simulink model "labsetup_cantonisim_distributed_periodic"  (R2019a)
settings: Solver=FixedStepDiscrete  StartTime=0.0  StopTime=1000  FixedStep=h  RelTol=1e-3
InitFcn:
  | ini_cantonisim_distributed
values from neighbouring files (symbols this model uses):
  C1 = [1 0]    [cantoni_LMI_labsetup.m]    (also in distributed_workspace_bak.mat)
  C2 = [0 1]    [cantoni_LMI_labsetup.m]    (also in distributed_workspace_bak.mat)
  ddelay = [0 0]    [distributed_workspace_bak.mat]
  h = legend(strcat('\phi(',plantTitle,')')); set(h,'FontSize',18)    [bodeJL.m]    (also in cantoni_LMI_labsetup.m = 1; distributed_workspace_bak.mat = 1)
  P1d = c2d(P1, h, 'zoh')    [cantoni_LMI_labsetup.m]
  P2d = c2d(P2, h, 'zoh')    [cantoni_LMI_labsetup.m]
  ss1d = c2d(ss1, h, 'tustin')    [cantoni_LMI_labsetup.m]
  ss2d = c2d(ss2, h, 'tustin')    [cantoni_LMI_labsetup.m]
  W1d = c2d(W1,h,'tustin')    [cantoni_LMI_labsetup.m]
  W2d = c2d(W2,h,'tustin')    [cantoni_LMI_labsetup.m]
undefined symbols (not defined in the file or in its folder): P3d, P4d, P5d, ss3d, ss4d, ss5d, W3d, W4d, W5d
settings Model: Creator=Jacob  LastModifiedBy=Jacob
settings SolverCC: AlgebraicLoopSolver=LineSearch
settings ModelReferenceCC: ModelReferenceMinAlgLoopOccurrences=on

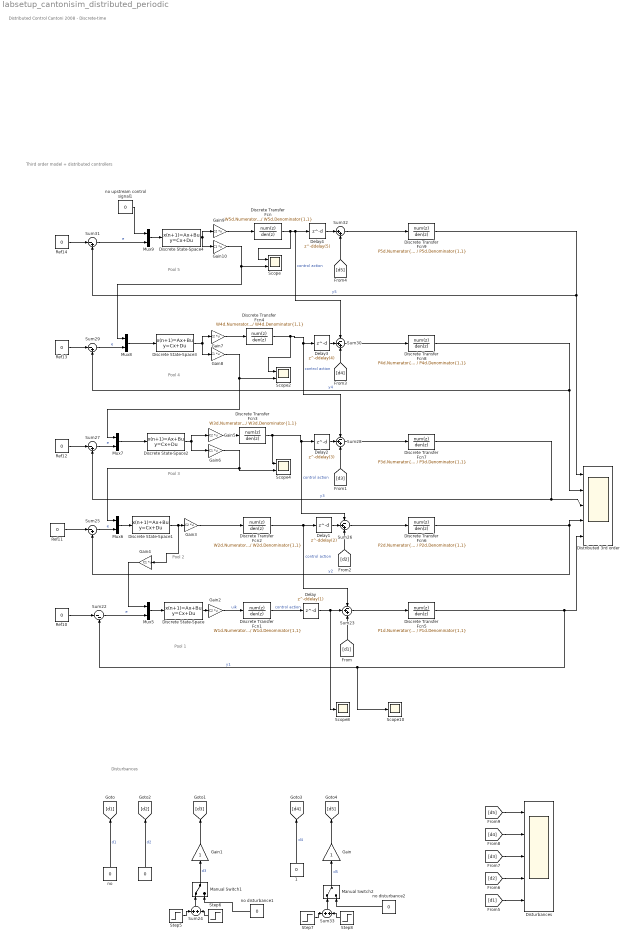
== system labsetup_cantonisim_distributed_periodic ==
  note: Disturbances
  note: Distributed Control Cantoni 2008 - Discrete-time
  note: Third order model + distributed controllers
  note: Pool 3
  note: Pool 5
  note: Pool 1
  note: Pool 2
  note: Pool 4
  " " : Constant  Value=0  SampleTime=h
  " 1" : Constant  Value=0  SampleTime=h
  Delay : Delay  DelayLength=ddelay(1)
  Delay1 : Delay  DelayLength=ddelay(2)
  Delay2 : Delay  DelayLength=ddelay(3)
  Delay3 : Delay  DelayLength=ddelay(4)
  Delay4 : Delay  DelayLength=ddelay(5)
  Discrete Transfer Fcn : DiscreteTransferFcn  Numerator=W5d.Numerator{1,1}  Denominator=W5d.Denominator{1,1}
  Discrete Transfer Fcn1 : DiscreteTransferFcn  Numerator=W1d.Numerator{1,1}  Denominator=W1d.Denominator{1,1}
  Discrete Transfer Fcn2 : DiscreteTransferFcn  Numerator=W2d.Numerator{1,1}  Denominator=W2d.Denominator{1,1}
  Discrete Transfer Fcn3 : DiscreteTransferFcn  Numerator=W3d.Numerator{1,1}  Denominator=W3d.Denominator{1,1}
  Discrete Transfer Fcn4 : DiscreteTransferFcn  Numerator=W4d.Numerator{1,1}  Denominator=W4d.Denominator{1,1}
  Discrete Transfer Fcn5 : DiscreteTransferFcn  Numerator=P1d.Numerator{1,1}  Denominator=P1d.Denominator{1,1}
  Discrete Transfer Fcn6 : DiscreteTransferFcn  Numerator=P2d.Numerator{1,1}  Denominator=P2d.Denominator{1,1}
  Discrete Transfer Fcn7 : DiscreteTransferFcn  Numerator=P3d.Numerator{1,1}  Denominator=P3d.Denominator{1,1}
  Discrete Transfer Fcn8 : DiscreteTransferFcn  Numerator=P4d.Numerator{1,1}  Denominator=P4d.Denominator{1,1}
  Discrete Transfer Fcn9 : DiscreteTransferFcn  Numerator=P5d.Numerator{1,1}  Denominator=P5d.Denominator{1,1}
  Discrete State-Space : DiscreteStateSpace  A=ss1d.A  B=ss1d.B  C=ss1d.C  D=ss1d.D  SampleTime=-1
  Discrete State-Space1 : DiscreteStateSpace  A=ss2d.A  B=ss2d.B  C=ss2d.C  D=ss2d.D  SampleTime=-1
  Discrete State-Space2 : DiscreteStateSpace  A=ss3d.A  B=ss3d.B  C=ss3d.C  D=ss3d.D  SampleTime=-1
  Discrete State-Space3 : DiscreteStateSpace  A=ss4d.A  B=ss4d.B  C=ss4d.C  D=ss4d.D  SampleTime=-1
  Discrete State-Space4 : DiscreteStateSpace  A=ss5d.A  B=ss5d.B  C=ss5d.C  D=ss5d.D  SampleTime=-1
  Distributed 3rd order : Scope  NumInputPorts=5
  Disturbances : Scope  NumInputPorts=5
  Gain : Gain
  Gain1 : Gain
  Gain{4,6,8,10} (4 alike) : Gain  Gain=C1  Multiplication=Matrix(K*u)
  Gain{2..3,5,7,9} (5 alike) : Gain  Gain=C2  Multiplication=Matrix(K*u)
  Manual Switch1 : ManualSwitch
  Manual Switch2 : ManualSwitch
  Mux{5..9} (5 alike) : Mux  Inputs=2
  Ref{10..14} (5 alike) : Constant  Value=0  SampleTime=h
  Scope : Scope  NumInputPorts=2
  Scope10 : Scope
  Scope2 : Scope  NumInputPorts=2
  Scope4 : Scope  NumInputPorts=2
  Scope8 : Scope
  Step5 : Step  Time=10  SampleTime=h
  Step6 : Step  Time=20  After=-1  SampleTime=h
  Step7 : Step  Time=100  SampleTime=h
  Step8 : Step  Time=150  After=-1  SampleTime=h
  Sum22 : Sum  Inputs=|--
  Sum{23,26,28,30} (4 alike) : Sum  Inputs=-++
  Sum24 : Sum  Inputs=+|+
  Sum{25,27,29,31} (4 alike) : Sum  Inputs=|-+
  Sum32 : Sum  Inputs=|++
  Sum33 : Sum  Inputs=+|+
  no : Constant  Value=0  SampleTime=h
  no disturbance1 : Constant  Value=0  SampleTime=h
  no disturbance2 : Constant  Value=0  SampleTime=h
  no upstream control signal1 : Constant  Value=0  SampleTime=h
  wires:
  Mux6/1 -> Discrete State-Space1/1
  Mux7/1 -> Discrete State-Space2/1
  Discrete Transfer Fcn4/1 -> Scope2/1, Delay3/1, Sum28/1  "control action"
  Mux5/1 -> Discrete State-Space/1
  Mux8/1 -> Discrete State-Space3/1
  [d2] -> Sum26/3
  Delay3/1 -> Sum30/2
  Discrete Transfer Fcn6/1 -> Sum25/2, Distributed 3rd order/4  "y2"
  Discrete Transfer Fcn8/1 -> Sum29/2, Distributed 3rd order/2  "y4"
  Discrete Transfer Fcn7/1 -> Sum27/2, Distributed 3rd order/3  "y3"
  Sum30/1 -> Discrete Transfer Fcn8/1
  Sum28/1 -> Discrete Transfer Fcn7/1
  Sum26/1 -> Discrete Transfer Fcn6/1
  Delay/1 -> Scope8/1, Sum23/2
  Sum22/1 -> Mux5/2  "e"
  Sum29/1 -> Mux8/2  "e"
  Sum31/1 -> Mux9/2  "e"
  Discrete Transfer Fcn9/1 -> Sum31/2, Distributed 3rd order/1  "y5"
  Delay1/1 -> Sum26/2
  Mux9/1 -> Discrete State-Space4/1
  [d3] -> Sum28/3
  Discrete Transfer Fcn5/1 -> Scope10/1, Sum22/2, Distributed 3rd order/5  "y1"
  Discrete Transfer Fcn1/1 -> Delay/1  "control action"
  Discrete Transfer Fcn2/1 -> Delay1/1, Sum23/1  "control action"
  Discrete Transfer Fcn3/1 -> Scope4/1, Delay2/1, Sum26/1  "control action"
  no upstream control signal1/1 -> Mux9/1
  Delay4/1 -> Sum32/1
  Ref13/1 -> Sum29/1
  Sum32/1 -> Discrete Transfer Fcn9/1
  Sum27/1 -> Mux7/2  "e"
  Ref10/1 -> Sum22/1
  Ref11/1 -> Sum25/1
  [d4] -> Sum30/3
  Ref14/1 -> Sum31/1
  Sum23/1 -> Discrete Transfer Fcn5/1
  Delay2/1 -> Sum28/2
  Ref12/1 -> Sum27/1
  Sum25/1 -> Mux6/2  "e"
  [d1] -> Sum23/3
  no disturbance1/1 -> Manual Switch1/2
  Step5/1 -> Sum24/1
  Sum24/1 -> Manual Switch1/1
  Step6/1 -> Sum24/2
  Manual Switch1/1 -> Gain1/1  "d3"
  " "/1 -> [d2]  "d2"
  " 1"/1 -> [d4]  "d4"
  Manual Switch2/1 -> Gain/1  "d5"
  [d5] -> Sum32/2
  no/1 -> [d1]  "d1"
  Step8/1 -> Sum33/2
  Sum33/1 -> Manual Switch2/1
  Step7/1 -> Sum33/1
  no disturbance2/1 -> Manual Switch2/2
  [d3] -> Disturbances/3
  [d1] -> Disturbances/5
  [d5] -> Disturbances/1
  [d2] -> Disturbances/4
  [d4] -> Disturbances/2
  Discrete State-Space/1 -> Gain2/1
  Discrete State-Space1/1 -> Gain3/1, Gain4/1
  Discrete State-Space2/1 -> Gain5/1, Gain6/1
  Gain6/1 -> Scope4/2, Mux6/1
  Discrete State-Space3/1 -> Gain7/1, Gain8/1
  Gain8/1 -> Scope2/2, Mux7/1
  Discrete State-Space4/1 -> Gain9/1, Gain10/1
  Gain10/1 -> Scope/2, Mux8/1
  Gain4/1 -> Mux5/1
  Gain2/1 -> Discrete Transfer Fcn1/1  "uik"
  Gain3/1 -> Discrete Transfer Fcn2/1
  Gain5/1 -> Discrete Transfer Fcn3/1
  Gain7/1 -> Discrete Transfer Fcn4/1
  Gain9/1 -> Discrete Transfer Fcn/1
  Discrete Transfer Fcn/1 -> Scope/1, Delay4/1, Sum30/1  "control action"
  Gain/1 -> [d5]
  Gain1/1 -> [d3]
